simulink model "Parametrica"  (R2020b)
settings: Solver=VariableStepAuto  StartTime=0.0  StopTime=Smi.general.simulation_time  FixedStep=0.001  MaxStep=0.001  RelTol=1e-3  AbsTol=1e-3  EnableMultiTasking=on
undefined symbols (not defined in the file or in its folder): Smi, X, Y, Z
libraries: sm_lib x755, nesl_utility x196, simulink x8, dspsrcs4 x8, cstblocks x8
(part 25 of 26)

== system Parametrica/MOVING CHASSIS/RR SUSPENSION/PUSHROD ==
  Cylindrical Solid : sm_lib/Body Elements/Cylindrical Solid  GraphicAmbientColor=[0.15 0.15 0.15 1.0]  BasedOnType=Density  CenterOfMass=[0 0 0]  CenterOfMassUnits=m  GraphicDiffuseColor=[0.8 0.6 0.0]  CylinderLength=Smi.Car.REAR.RIGHT.Dimension.Pushrod  CylinderLengthUnits=mm  CylinderRadius=Smi.Graphic.radius_links  CylinderRadiusUnits=mm  Density=1000  DensityUnits=kg/m^3  DoExposeReferenceFrame=off  GraphicEmissiveColor=[0.0 0.0 0.0 1.0]  ExportEntireGeometry=off  SerializedFrames=<Frames><Frame><Id>Frame1</Id><Value><Name>F1</Name><Origin><Source>GeometricFeature</Source><FeatureName>top surface</FeatureName></Origin><PrimaryAxis><DefinedDirection>+Z</DefinedDirection><Source>ReferenceFrame</Source><SourceDirection>+Z</SourceDirection><FeatureName></FeatureName></PrimaryAxis><SecondaryAxis><DefinedDirection>+X</DefinedDirection><Source>ReferenceFrame</Source><SourceDirection>+X</SourceDirection><FeatureName></FeatureName></SecondaryAxis></Value></Frame><Frame><Id>Frame2</Id><Value><Name>F2</Name><Origin><Source>GeometricFeature</Source><FeatureName>bottom curve</FeatureName></Origin><PrimaryAxis><DefinedDirection>+Z</DefinedDirection><Source>ReferenceFrame</Source><SourceDirection>+Z</SourceDirection><FeatureName></FeatureName></PrimaryAxis><SecondaryAxis><DefinedDirection>+X</DefinedDirection><Source>ReferenceFrame</Source><SourceDirection>+X</SourceDirection><FeatureName></FeatureName></SecondaryAxis></Value></Frame></Frames>  MarkerShape=Sphere  MarkerSize=10  GraphicType=FromGeometry  InertiaType=CalculateFromGeometry  Mass=1  MassUnits=kg  MomentsOfInertia=[1 1 1]  MomentsOfInertiaUnits=kg*m^2  GraphicOpacity=1.0  ProductsOfInertia=[0 0 0]  ProductsOfInertiaUnits=kg*m^2  GraphicShininess=75  GraphicSpecularColor=[0.5 0.5 0.5 1.0]  GraphicVisPropType=SimpleVisualProperties
  Spherical Solid : sm_lib/Body Elements/Spherical Solid  GraphicAmbientColor=[0.15 0.15 0.15 1.0]  BasedOnType=Density  CenterOfMass=[0 0 0]  CenterOfMassUnits=m  GraphicDiffuseColor=[0.8 0.6 0.0]  Density=0  DensityUnits=kg/m^3  DoExposeReferenceFrame=on  GraphicEmissiveColor=[0.0 0.0 0.0 1.0]  ExportEntireGeometry=off  SerializedExposedGeometries=<ExposedGeometries/>  SerializedFrames=<Frames/>  MarkerShape=Sphere  MarkerSize=10  GraphicType=FromGeometry  InertiaType=CalculateFromGeometry  Mass=1  MassUnits=kg  MomentsOfInertia=[1 1 1]  MomentsOfInertiaUnits=kg*m^2  GraphicOpacity=1.0  ProductsOfInertia=[0 0 0]  ProductsOfInertiaUnits=kg*m^2  GraphicShininess=75  GraphicSpecularColor=[0.5 0.5 0.5 1.0]  SphereRadius=Smi.Graphic.radius_spheres  SphereRadiusUnits=mm  GraphicVisPropType=SimpleVisualProperties
  Spherical Solid1 : sm_lib/Body Elements/Spherical Solid  GraphicAmbientColor=[0.15 0.15 0.15 1.0]  BasedOnType=Density  CenterOfMass=[0 0 0]  CenterOfMassUnits=m  GraphicDiffuseColor=[0.8 0.6 0.0]  Density=0  DensityUnits=kg/m^3  DoExposeReferenceFrame=on  GraphicEmissiveColor=[0.0 0.0 0.0 1.0]  ExportEntireGeometry=off  SerializedExposedGeometries=<ExposedGeometries/>  SerializedFrames=<Frames/>  MarkerShape=Sphere  MarkerSize=10  GraphicType=FromGeometry  InertiaType=CalculateFromGeometry  Mass=1  MassUnits=kg  MomentsOfInertia=[1 1 1]  MomentsOfInertiaUnits=kg*m^2  GraphicOpacity=1.0  ProductsOfInertia=[0 0 0]  ProductsOfInertiaUnits=kg*m^2  GraphicShininess=75  GraphicSpecularColor=[0.5 0.5 0.5 1.0]  SphereRadius=Smi.Graphic.radius_spheres  SphereRadiusUnits=mm  GraphicVisPropType=SimpleVisualProperties
  CRANK : PMIOPort  Side=Left
  UPPER WISHBONE : PMIOPort  Port=2  Side=Right
  connections:
  Cylindrical Solid/RConn1 -- Spherical Solid/RConn1 -- CRANK/RConn1
  Spherical Solid1/RConn1 -- UPPER WISHBONE/RConn1 -- Cylindrical Solid/LConn1

== system Parametrica/MOVING CHASSIS/RR SUSPENSION/STEM ==
  ATTACCO STEM : sm_lib/Body Elements/Extruded Solid  GraphicAmbientColor=[0.15 0.15 0.15 1.0]  BasedOnType=Density  CenterOfMass=[0 0 0]  CenterOfMassUnits=m  GraphicDiffuseColor=[1.0 0.0 0.2]  ExportConvexHullGeometry=off  ExtrusionCrossSection=[0 0; 22 0; 20 22; 2 22]  ExtrusionCrossSectionUnits=mm  Density=1000  DensityUnits=kg/m^3  DoExposeReferenceFrame=off  GraphicEmissiveColor=[0.0 0.0 0.0 1.0]  ExportEntireGeometry=off  ExtrusionLength=5  ExtrusionLengthUnits=mm  ExtrusionType=General  SerializedFrames=<Frames><Frame><Id>Frame1</Id><Value><Name>F1</Name><Origin><Source>GeometricFeature</Source><FeatureName>side surface 1</FeatureName></Origin><PrimaryAxis><DefinedDirection>+Z</DefinedDirection><Source>ReferenceFrame</Source><SourceDirection>+Y</SourceDirection><FeatureName></FeatureName></PrimaryAxis><SecondaryAxis><DefinedDirection>+X</DefinedDirection><Source>ReferenceFrame</Source><SourceDirection>+X</SourceDirection><FeatureName></FeatureName></SecondaryAxis></Value></Frame><Frame><Id>Frame2</Id><Value><Name>F2</Name><Origin><Source>CenterOfMassFrame</Source><FeatureName></FeatureName></Origin><PrimaryAxis><DefinedDirection>+Y</DefinedDirection><Source>ReferenceFrame</Source><SourceDirection>-Y</SourceDirection><FeatureName></FeatureName></PrimaryAxis><SecondaryAxis><DefinedDirection>+X</DefinedDirection><Source>ReferenceFrame</Source><SourceDirection>+X</SourceDirection><FeatureName></FeatureName></SecondaryAxis></Value></Frame></Frames>  MarkerShape=Sphere  MarkerSize=10  GraphicType=FromGeometry  InertiaType=CalculateFromGeometry  Mass=1  MassUnits=kg  MomentsOfInertia=[1 1 1]  MomentsOfInertiaUnits=kg*m^2  PolygonNumSides=3  GraphicOpacity=1.0  PolygonOuterRadius=1  PolygonOuterRadiusUnits=m  ProductsOfInertia=[0 0 0]  ProductsOfInertiaUnits=kg*m^2  GraphicShininess=75  GraphicSpecularColor=[0.5 0.5 0.5 1.0]  GraphicVisPropType=SimpleVisualProperties
  STEM : sm_lib/Body Elements/Revolved Solid  GraphicAmbientColor=[0.15 0.15 0.15 1.0]  BasedOnType=Density  CenterOfMass=[0 0 0]  CenterOfMassUnits=m  GraphicDiffuseColor=[1.0 0.0 0.2]  ExportConvexHullGeometry=off  Density=1000  DensityUnits=kg/m^3  DoExposeReferenceFrame=on  GraphicEmissiveColor=[0.0 0.0 0.0 1.0]  ExportEntireGeometry=off  SerializedFrames=<Frames><Frame><Id>Frame1</Id><Value><Name>F1</Name><Origin><Source>GeometricFeature</Source><FeatureName>side surface 5</FeatureName></Origin><PrimaryAxis><DefinedDirection>+Z</DefinedDirection><Source>ReferenceFrame</Source><SourceDirection>+Z</SourceDirection><FeatureName></FeatureName></PrimaryAxis><SecondaryAxis><DefinedDirection>+X</DefinedDirection><Source>ReferenceFrame</Source><SourceDirection>+X</SourceDirection><FeatureName></FeatureName></SecondaryAxis></Value></Frame></Frames>  MarkerShape=Sphere  MarkerSize=10  GraphicType=FromGeometry  InertiaType=CalculateFromGeometry  Mass=1  MassUnits=kg  MomentsOfInertia=[1 1 1]  MomentsOfInertiaUnits=kg*m^2  GraphicOpacity=1.0  ProductsOfInertia=[0 0 0]  ProductsOfInertiaUnits=kg*m^2  RevolutionCrossSection=[0 0 ; 3 0 ; 3 50 ; 21 50 ; 21 52 ; 0 52]  RevolutionCrossSectionUnits=mm  RevolutionAngle=180  RevolutionAngleUnits=deg  RevolutionExtent=Full  GraphicShininess=75  GraphicSpecularColor=[0.5 0.5 0.5 1.0]  GraphicVisPropType=SimpleVisualProperties
  CRANK : PMIOPort  Side=Left
  AMMO : PMIOPort  Port=2  Side=Right
  connections:
  ATTACCO STEM/LConn1 -- STEM/LConn1
  ATTACCO STEM/RConn1 -- CRANK/RConn1
  STEM/RConn1 -- AMMO/RConn1

== system Parametrica/MOVING CHASSIS/RR SUSPENSION/TIE ROD ==
  Cylindrical Solid : sm_lib/Body Elements/Cylindrical Solid  GraphicAmbientColor=[0.15 0.15 0.15 1.0]  BasedOnType=Density  CenterOfMass=[0 0 0]  CenterOfMassUnits=m  GraphicDiffuseColor=[1.0 0.6 0.4]  CylinderLength=Smi.Car.REAR.RIGHT.Dimension.Tie_rod  CylinderLengthUnits=mm  CylinderRadius=Smi.Graphic.radius_links  CylinderRadiusUnits=mm  Density=1000  DensityUnits=kg/m^3  DoExposeReferenceFrame=off  GraphicEmissiveColor=[0.0 0.0 0.0 1.0]  ExportEntireGeometry=off  SerializedFrames=<Frames><Frame><Id>Frame1</Id><Value><Name>F1</Name><Origin><Source>GeometricFeature</Source><FeatureName>top surface</FeatureName></Origin><PrimaryAxis><DefinedDirection>+Z</DefinedDirection><Source>ReferenceFrame</Source><SourceDirection>+Z</SourceDirection><FeatureName></FeatureName></PrimaryAxis><SecondaryAxis><DefinedDirection>+X</DefinedDirection><Source>ReferenceFrame</Source><SourceDirection>+X</SourceDirection><FeatureName></FeatureName></SecondaryAxis></Value></Frame><Frame><Id>Frame2</Id><Value><Name>F2</Name><Origin><Source>GeometricFeature</Source><FeatureName>bottom curve</FeatureName></Origin><PrimaryAxis><DefinedDirection>+Z</DefinedDirection><Source>ReferenceFrame</Source><SourceDirection>+Z</SourceDirection><FeatureName></FeatureName></PrimaryAxis><SecondaryAxis><DefinedDirection>+X</DefinedDirection><Source>ReferenceFrame</Source><SourceDirection>+X</SourceDirection><FeatureName></FeatureName></SecondaryAxis></Value></Frame></Frames>  MarkerShape=Sphere  MarkerSize=10  GraphicType=FromGeometry  InertiaType=CalculateFromGeometry  Mass=1  MassUnits=kg  MomentsOfInertia=[1 1 1]  MomentsOfInertiaUnits=kg*m^2  GraphicOpacity=1.0  ProductsOfInertia=[0 0 0]  ProductsOfInertiaUnits=kg*m^2  GraphicShininess=75  GraphicSpecularColor=[0.5 0.5 0.5 1.0]  GraphicVisPropType=SimpleVisualProperties
  Spherical Solid : sm_lib/Body Elements/Spherical Solid  GraphicAmbientColor=[0.15 0.15 0.15 1.0]  BasedOnType=Density  CenterOfMass=[0 0 0]  CenterOfMassUnits=m  GraphicDiffuseColor=[1.0 0.6 0.4]  Density=0  DensityUnits=kg/m^3  DoExposeReferenceFrame=on  GraphicEmissiveColor=[0.0 0.0 0.0 1.0]  ExportEntireGeometry=off  SerializedExposedGeometries=<ExposedGeometries/>  SerializedFrames=<Frames/>  MarkerShape=Sphere  MarkerSize=10  GraphicType=FromGeometry  InertiaType=CalculateFromGeometry  Mass=1  MassUnits=kg  MomentsOfInertia=[1 1 1]  MomentsOfInertiaUnits=kg*m^2  GraphicOpacity=1.0  ProductsOfInertia=[0 0 0]  ProductsOfInertiaUnits=kg*m^2  GraphicShininess=75  GraphicSpecularColor=[0.5 0.5 0.5 1.0]  SphereRadius=Smi.Graphic.radius_spheres  SphereRadiusUnits=mm  GraphicVisPropType=SimpleVisualProperties
  Spherical Solid1 : sm_lib/Body Elements/Spherical Solid  GraphicAmbientColor=[0.15 0.15 0.15 1.0]  BasedOnType=Density  CenterOfMass=[0 0 0]  CenterOfMassUnits=m  GraphicDiffuseColor=[1.0 0.6 0.4]  Density=0  DensityUnits=kg/m^3  DoExposeReferenceFrame=on  GraphicEmissiveColor=[0.0 0.0 0.0 1.0]  ExportEntireGeometry=off  SerializedExposedGeometries=<ExposedGeometries/>  SerializedFrames=<Frames/>  MarkerShape=Sphere  MarkerSize=10  GraphicType=FromGeometry  InertiaType=CalculateFromGeometry  Mass=1  MassUnits=kg  MomentsOfInertia=[1 1 1]  MomentsOfInertiaUnits=kg*m^2  GraphicOpacity=1.0  ProductsOfInertia=[0 0 0]  ProductsOfInertiaUnits=kg*m^2  GraphicShininess=75  GraphicSpecularColor=[0.5 0.5 0.5 1.0]  SphereRadius=Smi.Graphic.radius_spheres  SphereRadiusUnits=mm  GraphicVisPropType=SimpleVisualProperties
  TIE HUB : PMIOPort  Side=Left
  TIE RACK : PMIOPort  Port=2  Side=Right
  connections:
  Cylindrical Solid/RConn1 -- Spherical Solid/RConn1 -- TIE RACK/RConn1
  Spherical Solid1/RConn1 -- TIE HUB/RConn1 -- Cylindrical Solid/LConn1

== system Parametrica/MOVING CHASSIS/RR SUSPENSION/UPPER WISHBONE ==
  A : sm_lib/Body Elements/Spherical Solid  GraphicAmbientColor=[0.15 0.15 0.15 1.0]  BasedOnType=Density  CenterOfMass=[0 0 0]  CenterOfMassUnits=m  GraphicDiffuseColor=[1.0 0.6 0.2]  Density=0  DensityUnits=kg/m^3  DoExposeReferenceFrame=on  GraphicEmissiveColor=[0.0 0.0 0.0 1.0]  ExportEntireGeometry=off  SerializedExposedGeometries=<ExposedGeometries/>  SerializedFrames=<Frames/>  MarkerShape=Sphere  MarkerSize=10  GraphicType=FromGeometry  InertiaType=CalculateFromGeometry  Mass=1  MassUnits=kg  MomentsOfInertia=[1 1 1]  MomentsOfInertiaUnits=kg*m^2  GraphicOpacity=1.0  ProductsOfInertia=[0 0 0]  ProductsOfInertiaUnits=kg*m^2  GraphicShininess=75  GraphicSpecularColor=[0.5 0.5 0.5 1.0]  SphereRadius=Smi.Graphic.radius_spheres  SphereRadiusUnits=mm  GraphicVisPropType=SimpleVisualProperties
  A-B : sm_lib/Frames and Transforms/Rigid Transform  TranslationMethod=None  TranslationStandardOffset=0  TranslationLengthUnit=mm  TranslationStandardAxis=+Z  TranslationCartesianOffset=Smi.Car.FRONT.LEFT.A  TranslationROffset=0  TranslationROffsetUnits=m  TranslationZOffset=0  TranslationZOffsetUnits=m  TranslationThetaOffset=0  TranslationThetaOffsetUnits=deg  RotationMethod=StandardAxis  RotationAngleUnits=rad  RotationStandardAxis=+Z  RotationAngle=-Smi.Car.REAR.RIGHT.Dimension.plane_UW.wish_angle  RotationArbitraryAxis=[0 0 1]  FollAlignAxisA=+X  BaseAlignAxisA=+Y  FollAlignAxisB=+Y  BaseAlignAxisB=+Z  RotationSequenceAxes=FollowerAxes  RotationSequence=XYZ  RotationSequenceAngles=0  RotationSequenceAnglesUnits=rad  RotationMatrix=[1 0 0; 0 1 0; 0 0 1]
      settings: SourceProductName=Multibody
  A-PS : sm_lib/Frames and Transforms/Rigid Transform  TranslationMethod=Cartesian  TranslationStandardOffset=0  TranslationLengthUnit=mm  TranslationStandardAxis=+Z  TranslationCartesianOffset=Smi.Car.REAR.RIGHT.Dimension.plane_UW.PS_t_coord-Smi.Car.REAR.RIGHT.Dimension.plane_UW.A_t_coord  TranslationROffset=0  TranslationROffsetUnits=m  TranslationZOffset=0  TranslationZOffsetUnits=m  TranslationThetaOffset=0  TranslationThetaOffsetUnits=deg  RotationMethod=None  RotationAngleUnits=deg  RotationStandardAxis=+Z  RotationAngle=0.0  RotationArbitraryAxis=[0 0 1]  FollAlignAxisA=+X  BaseAlignAxisA=+Y  FollAlignAxisB=+Y  BaseAlignAxisB=+Z  RotationSequenceAxes=FollowerAxes  RotationSequence=XYZ  RotationSequenceAngles=0  RotationSequenceAnglesUnits=rad  RotationMatrix=[1 0 0; 0 1 0; 0 0 1]
      settings: SourceProductName=Multibody
  B : sm_lib/Body Elements/Spherical Solid  GraphicAmbientColor=[0.15 0.15 0.15 1.0]  BasedOnType=Density  CenterOfMass=[0 0 0]  CenterOfMassUnits=m  GraphicDiffuseColor=[1.0 0.6 0.2]  Density=0  DensityUnits=kg/m^3  DoExposeReferenceFrame=on  GraphicEmissiveColor=[0.0 0.0 0.0 1.0]  ExportEntireGeometry=off  SerializedExposedGeometries=<ExposedGeometries/>  SerializedFrames=<Frames/>  MarkerShape=Sphere  MarkerSize=10  GraphicType=FromGeometry  InertiaType=CalculateFromGeometry  Mass=1  MassUnits=kg  MomentsOfInertia=[1 1 1]  MomentsOfInertiaUnits=kg*m^2  GraphicOpacity=1.0  ProductsOfInertia=[0 0 0]  ProductsOfInertiaUnits=kg*m^2  GraphicShininess=75  GraphicSpecularColor=[0.5 0.5 0.5 1.0]  SphereRadius=Smi.Graphic.radius_spheres  SphereRadiusUnits=mm  GraphicVisPropType=SimpleVisualProperties
  INNER CYL : sm_lib/Body Elements/Cylindrical Solid  GraphicAmbientColor=[0.15 0.15 0.15 1.0]  BasedOnType=Density  CenterOfMass=[0 0 0]  CenterOfMassUnits=m  GraphicDiffuseColor=[1.0 0.6 0.2]  CylinderLength=Smi.Car.REAR.RIGHT.Dimension.inner_cyl_UW  CylinderLengthUnits=mm  CylinderRadius=Smi.Graphic.radius_links  CylinderRadiusUnits=mm  Density=1000  DensityUnits=kg/m^3  DoExposeReferenceFrame=off  GraphicEmissiveColor=[0.0 0.0 0.0 1.0]  ExportEntireGeometry=off  SerializedFrames=<Frames><Frame><Id>Frame3</Id><Value><Name>F1</Name><Origin><Source>GeometricFeature</Source><FeatureName>top curve</FeatureName></Origin><PrimaryAxis><DefinedDirection>+Z</DefinedDirection><Source>ReferenceFrame</Source><SourceDirection>+Y</SourceDirection><FeatureName></FeatureName></PrimaryAxis><SecondaryAxis><DefinedDirection>+X</DefinedDirection><Source>ReferenceFrame</Source><SourceDirection>+X</SourceDirection><FeatureName></FeatureName></SecondaryAxis></Value></Frame><Frame><Id>Frame4</Id><Value><Name>F4</Name><Origin><Source>GeometricFeature</Source><FeatureName>bottom surface</FeatureName></Origin><PrimaryAxis><DefinedDirection>+Z</DefinedDirection><Source>ReferenceFrame</Source><SourceDirection>+X</SourceDirection><FeatureName></FeatureName></PrimaryAxis><SecondaryAxis><DefinedDirection>+X</DefinedDirection><Source>ReferenceFrame</Source><SourceDirection>+Y</SourceDirection><FeatureName></FeatureName></SecondaryAxis></Value></Frame></Frames>  MarkerShape=Sphere  MarkerSize=10  GraphicType=FromGeometry  InertiaType=CalculateFromGeometry  Mass=1  MassUnits=kg  MomentsOfInertia=[1 1 1]  MomentsOfInertiaUnits=kg*m^2  GraphicOpacity=1.0  ProductsOfInertia=[0 0 0]  ProductsOfInertiaUnits=kg*m^2  GraphicShininess=75  GraphicSpecularColor=[0.5 0.5 0.5 1.0]  GraphicVisPropType=SimpleVisualProperties
  OUTER CYL : sm_lib/Body Elements/Cylindrical Solid  GraphicAmbientColor=[0.15 0.15 0.15 1.0]  BasedOnType=Density  CenterOfMass=[0 0 0]  CenterOfMassUnits=m  GraphicDiffuseColor=[1.0 0.6 0.2]  CylinderLength=Smi.Car.REAR.RIGHT.Dimension.outer_cyl_UW  CylinderLengthUnits=mm  CylinderRadius=Smi.Graphic.radius_links  CylinderRadiusUnits=mm  Density=1000  DensityUnits=kg/m^3  DoExposeReferenceFrame=off  GraphicEmissiveColor=[0.0 0.0 0.0 1.0]  ExportEntireGeometry=off  SerializedFrames=<Frames><Frame><Id>Frame1</Id><Value><Name>F1</Name><Origin><Source>GeometricFeature</Source><FeatureName>top surface</FeatureName></Origin><PrimaryAxis><DefinedDirection>+Y</DefinedDirection><Source>ReferenceFrame</Source><SourceDirection>+Z</SourceDirection><FeatureName></FeatureName></PrimaryAxis><SecondaryAxis><DefinedDirection>+X</DefinedDirection><Source>ReferenceFrame</Source><SourceDirection>+X</SourceDirection><FeatureName></FeatureName></SecondaryAxis></Value></Frame><Frame><Id>Frame2</Id><Value><Name>F2</Name><Origin><Source>GeometricFeature</Source><FeatureName>bottom surface</FeatureName></Origin><PrimaryAxis><DefinedDirection>+Y</DefinedDirection><Source>ReferenceFrame</Source><SourceDirection>+Z</SourceDirection><FeatureName></FeatureName></PrimaryAxis><SecondaryAxis><DefinedDirection>+X</DefinedDirection><Source>ReferenceFrame</Source><SourceDirection>+X</SourceDirection><FeatureName></FeatureName></SecondaryAxis></Value></Frame></Frames>  MarkerShape=Sphere  MarkerSize=10  GraphicType=FromGeometry  InertiaType=CalculateFromGeometry  Mass=1  MassUnits=kg  MomentsOfInertia=[1 1 1]  MomentsOfInertiaUnits=kg*m^2  GraphicOpacity=1.0  ProductsOfInertia=[0 0 0]  ProductsOfInertiaUnits=kg*m^2  GraphicShininess=75  GraphicSpecularColor=[0.5 0.5 0.5 1.0]  GraphicVisPropType=SimpleVisualProperties
  UBJ : sm_lib/Body Elements/Spherical Solid  GraphicAmbientColor=[0.15 0.15 0.15 1.0]  BasedOnType=Density  CenterOfMass=[0 0 0]  CenterOfMassUnits=m  GraphicDiffuseColor=[1.0 0.6 0.2]  Density=1000  DensityUnits=kg/m^3  DoExposeReferenceFrame=on  GraphicEmissiveColor=[0.0 0.0 0.0 1.0]  ExportEntireGeometry=off  SerializedExposedGeometries=<ExposedGeometries/>  SerializedFrames=<Frames/>  MarkerShape=Sphere  MarkerSize=10  GraphicType=FromGeometry  InertiaType=CalculateFromGeometry  Mass=1  MassUnits=kg  MomentsOfInertia=[1 1 1]  MomentsOfInertiaUnits=kg*m^2  GraphicOpacity=1.0  ProductsOfInertia=[0 0 0]  ProductsOfInertiaUnits=kg*m^2  GraphicShininess=75  GraphicSpecularColor=[0.5 0.5 0.5 1.0]  SphereRadius=Smi.Graphic.radius_spheres  SphereRadiusUnits=mm  GraphicVisPropType=SimpleVisualProperties
  A UCS : PMIOPort  Side=Left
  B UCS : PMIOPort  Port=2  Side=Left
  PUSHROD UCS : PMIOPort  Port=3  Side=Right
  UBJ UCS : PMIOPort  Port=4  Side=Right
  connections:
  A UCS/RConn1 -- OUTER CYL/RConn1 -- A-PS/LConn1 -- A/RConn1
  UBJ UCS/RConn1 -- UBJ/RConn1 -- OUTER CYL/LConn1 -- A-B/LConn1
  B UCS/RConn1 -- B/RConn1 -- INNER CYL/LConn1
  A-B/RConn1 -- INNER CYL/RConn1
  A-PS/RConn1 -- PUSHROD UCS/RConn1

== system Parametrica/MOVING CHASSIS/RR SUSPENSION/WHEEL ==
  Revolved Solid : sm_lib/Body Elements/Revolved Solid  Commented=on  GraphicAmbientColor=[0.15 0.15 0.15 1.0]  BasedOnType=Density  CenterOfMass=[0 0 0]  CenterOfMassUnits=m  GraphicDiffuseColor=[0.8 1.0 0.8]  ExportConvexHullGeometry=off  Density=1000  DensityUnits=kg/m^3  DoExposeReferenceFrame=off  GraphicEmissiveColor=[0.0 0.0 0.0 1.0]  ExportEntireGeometry=off  SerializedFrames=<Frames><Frame><Id>Frame1</Id><Value><Name>F1</Name><Origin><Source>ReferenceFrame</Source><FeatureName></FeatureName></Origin><PrimaryAxis><DefinedDirection>+Z</DefinedDirection><Source>ReferenceFrame</Source><SourceDirection>+Y</SourceDirection><FeatureName></FeatureName></PrimaryAxis><SecondaryAxis><DefinedDirection>+X</DefinedDirection><Source>ReferenceFrame</Source><SourceDirection>-X</SourceDirection><FeatureName></FeatureName></SecondaryAxis></Value></Frame></Frames>  MarkerShape=Sphere  MarkerSize=10  GraphicType=FromGeometry  InertiaType=CalculateFromGeometry  Mass=1  MassUnits=kg  MomentsOfInertia=[1 1 1]  MomentsOfInertiaUnits=kg*m^2  GraphicOpacity=0.5  ProductsOfInertia=[0 0 0]  ProductsOfInertiaUnits=kg*m^2  RevolutionCrossSection=Smi.Car.FRONT.LEFT.Dimension.tyre_profile  RevolutionCrossSectionUnits=mm  RevolutionAngle=180  RevolutionAngleUnits=deg  RevolutionExtent=Full  GraphicShininess=75  GraphicSpecularColor=[0.5 0.5 0.5 1.0]  GraphicVisPropType=SimpleVisualProperties
  Rigid Transform : sm_lib/Frames and Transforms/Rigid Transform  TranslationMethod=StandardAxis  TranslationStandardOffset=Smi.Car.REAR.RIGHT.TYRE_DIAMETER/2+3  TranslationLengthUnit=mm  TranslationStandardAxis=-Z  TranslationCartesianOffset=[0 0 0]  TranslationROffset=0  TranslationROffsetUnits=m  TranslationZOffset=0  TranslationZOffsetUnits=m  TranslationThetaOffset=0  TranslationThetaOffsetUnits=deg  RotationMethod=None  RotationAngleUnits=deg  RotationStandardAxis=+Z  RotationAngle=0.0  RotationArbitraryAxis=[0 0 1]  FollAlignAxisA=+X  BaseAlignAxisA=+Y  FollAlignAxisB=+Y  BaseAlignAxisB=+Z  RotationSequenceAxes=FollowerAxes  RotationSequence=XYX  RotationSequenceAngles=[0 0 0]  RotationSequenceAnglesUnits=deg  RotationMatrix=[1 0 0; 0 1 0; 0 0 1]
  Spherical Solid : sm_lib/Body Elements/Spherical Solid  Commented=on  GraphicAmbientColor=[0.15 0.15 0.15 1.0]  BasedOnType=Density  CenterOfMass=[0 0 0]  CenterOfMassUnits=m  GraphicDiffuseColor=[1.0 0.0 0.2]  Density=0  DensityUnits=kg/m^3  DoExposeReferenceFrame=on  GraphicEmissiveColor=[0.0 0.0 0.0 1.0]  ExportEntireGeometry=on  SerializedExposedGeometries=<ExposedGeometries><ExposedGeometry><RawGeometryId>entire</RawGeometryId><ExposedGeometryId>G</ExposedGeometryId></ExposedGeometry></ExposedGeometries>  SerializedFrames=<Frames/>  MarkerShape=Sphere  MarkerSize=10  GraphicType=FromGeometry  InertiaType=CalculateFromGeometry  Mass=1  MassUnits=kg  MomentsOfInertia=[1 1 1]  MomentsOfInertiaUnits=kg*m^2  GraphicOpacity=0  ProductsOfInertia=[0 0 0]  ProductsOfInertiaUnits=kg*m^2  GraphicShininess=75  GraphicSpecularColor=[0.5 0.5 0.5 1.0]  SphereRadius=Smi.Car.FRONT.LEFT.TYRE_DIAMETER/2  SphereRadiusUnits=mm  GraphicVisPropType=SimpleVisualProperties
  TIRE : sm_lib/Body Elements/File Solid  ExtGeomFileName=Parameters\tire.stp  UnitType=FromFile  ExtGeomFileUnits=m  StepReaderType=HEX  ExportConvexHullGeometry=on  InertiaType=PointMass  Mass=1  MassUnits=kg  CenterOfMass=[0 0 0]  CenterOfMassUnits=m  MomentsOfInertia=[1 1 1]  MomentsOfInertiaUnits=kg*m^2  ProductsOfInertia=[0 0 0]  ProductsOfInertiaUnits=kg*m^2  BasedOnType=DensityFromFile  Density=1000  DensityUnits=kg/m^3  DoExposeReferenceFrame=off  SerializedFrames=<Frames><Frame><Id>Frame1</Id><Value><Name>F1</Name><Origin><Source>ReferenceFrame</Source><FeatureName></FeatureName></Origin><PrimaryAxis><DefinedDirection>+Z</DefinedDirection><Source>ReferenceFrame</Source><SourceDirection>+Z</SourceDirection><FeatureName></FeatureName></PrimaryAxis><SecondaryAxis><DefinedDirection>+X</DefinedDirection><Source>ReferenceFrame</Source><SourceDirection>+Y</SourceDirection><FeatureName></FeatureName></SecondaryAxis></Value></Frame></Frames>  GraphicType=FromGeometry  MarkerShape=Sphere  MarkerSize=10  GraphicVisPropType=SimpleVisualProperties  GraphicDiffuseColor=[0.5 0.5 0.5]  GraphicSpecularColor=[0.5 0.5 0.5 1.0]  GraphicAmbientColor=[0.15 0.15 0.15 1.0]  GraphicEmissiveColor=[0.0 0.0 0.0 1.0]  GraphicShininess=75  GraphicOpacity=1.0
  WC : PMIOPort  Side=Left
  Contact Sphere : PMIOPort  Port=2  Side=Right
  CP REAL : PMIOPort  Port=3  Side=Right
  connections:
  Spherical Solid/RConn1 -- Rigid Transform/LConn1 -- TIRE/LConn1 -- WC/RConn1
  CP REAL/RConn1 -- Rigid Transform/RConn1
  Contact Sphere/RConn1 -- TIRE/RConn1

== system Parametrica/MOVING CHASSIS/RR SUSPENSION/Wheel Angle Sensing ==
  Gain : Gain  Gain=-1
  PS-Simulink Converter : nesl_utility/PS-Simulink Converter  PhysicalDomain=network_engine_domain  SubClassName=ps_output  LeftPortType=input  RightPortType=output  PseudoPeriodic=off  Frequencies=[]  Unit=deg  AffineConversion=off
  PS-Simulink Converter1 : nesl_utility/PS-Simulink Converter  PhysicalDomain=network_engine_domain  SubClassName=ps_output  LeftPortType=input  RightPortType=output  PseudoPeriodic=off  Frequencies=[]  Unit=inherit  AffineConversion=off
  PS-Simulink Converter2 : nesl_utility/PS-Simulink Converter  PhysicalDomain=network_engine_domain  SubClassName=ps_output  LeftPortType=input  RightPortType=output  PseudoPeriodic=off  Frequencies=[]  Unit=deg  AffineConversion=off
  PS-Simulink Converter3 : nesl_utility/PS-Simulink Converter  PhysicalDomain=network_engine_domain  SubClassName=ps_output  LeftPortType=input  RightPortType=output  PseudoPeriodic=off  Frequencies=[]  Unit=inherit  AffineConversion=off
  Product : Product
  Product1 : Product
  Scope : Scope
  Scope1 : Scope
  Selector : Selector  InputPortWidth=3  IndexOptions=Index vector (dialog)  Indices=[1]  OutputSizes=1
  Selector1 : Selector  InputPortWidth=3  IndexOptions=Index vector (dialog)  Indices=[3]  OutputSizes=1
  To Workspace : ToWorkspace  VariableName=RR_camber  SaveFormat=Timeseries  SampleTime=-1
  To Workspace1 : ToWorkspace  VariableName=RR_toe  SaveFormat=Timeseries  SampleTime=-1
  Transform Sensor : sm_lib/Frames and Transforms/Transform Sensor  MeasurementFrame=Base  SenseAngle=on  SenseAxis=on  SenseAngle1=off  SenseAngle2=off  SenseAngle3=off  SenseQ=off  SenseR=off  SenseOmegaX=off  SenseOmegaY=off  SenseOmegaZ=off  SenseOmega1=off  SenseOmega2=off  SenseOmega3=off  SenseQDot=off  SenseRDot=off  SenseAlphaX=off  SenseAlphaY=off  SenseAlphaZ=off  SenseAlpha1=off  SenseAlpha2=off  SenseAlpha3=off  SenseQDDot=off  SenseRDDot=off  SenseX=off  SenseY=off  SenseZ=off  SenseRad=off  SenseAzim=off  SenseDist=off  SenseInc=off  SenseXDot=off  SenseYDot=off  SenseZDot=off  SenseRadDot=off  SenseAzimDot=off  SenseDistDot=off  SenseIncDot=off  SenseXDDot=off  SenseYDDot=off  SenseZDDot=off  SenseRadDDot=off  SenseAzimDDot=off  SenseDistDDot=off  SenseIncDDot=off
  Transform Sensor1 : sm_lib/Frames and Transforms/Transform Sensor  MeasurementFrame=Base  SenseAngle=on  SenseAxis=on  SenseAngle1=off  SenseAngle2=off  SenseAngle3=off  SenseQ=off  SenseR=off  SenseOmegaX=off  SenseOmegaY=off  SenseOmegaZ=off  SenseOmega1=off  SenseOmega2=off  SenseOmega3=off  SenseQDot=off  SenseRDot=off  SenseAlphaX=off  SenseAlphaY=off  SenseAlphaZ=off  SenseAlpha1=off  SenseAlpha2=off  SenseAlpha3=off  SenseQDDot=off  SenseRDDot=off  SenseX=off  SenseY=off  SenseZ=off  SenseRad=off  SenseAzim=off  SenseDist=off  SenseInc=off  SenseXDot=off  SenseYDot=off  SenseZDot=off  SenseRadDot=off  SenseAzimDot=off  SenseDistDot=off  SenseIncDot=off  SenseXDDot=off  SenseYDDot=off  SenseZDDot=off  SenseRadDDot=off  SenseAzimDDot=off  SenseDistDDot=off  SenseIncDDot=off
  WHEEL : PMIOPort  Side=Left
  WORLD : PMIOPort  Port=2  Side=Right
  wires:
  Product/1 -> To Workspace/1, Scope/1
  PS-Simulink Converter/1 -> Product/1
  Selector1/1 -> Product1/2
  PS-Simulink Converter2/1 -> Gain/1
  Selector/1 -> Product/2
  Product1/1 -> To Workspace1/1, Scope1/1
  PS-Simulink Converter1/1 -> Selector/1
  PS-Simulink Converter3/1 -> Selector1/1
  Gain/1 -> Product1/1
  connections:
  PS-Simulink Converter2/LConn1 -- Transform Sensor1/RConn2
  PS-Simulink Converter/LConn1 -- Transform Sensor/RConn2
  Transform Sensor/RConn1 -- Transform Sensor1/RConn1 -- WORLD/RConn1
  Transform Sensor1/LConn1 -- Transform Sensor/LConn1 -- WHEEL/RConn1
  PS-Simulink Converter3/LConn1 -- Transform Sensor1/RConn3
  PS-Simulink Converter1/LConn1 -- Transform Sensor/RConn3

== system Parametrica/FIXED CHASSIS/ACTUATOR FL/ACTUATOR IN//OUT/Random sine waves ==
  Clock : Clock
  Constant : Constant  Value=Smi.general.random_harshness
  Constant1 : Constant  Value=-100
  Divide : Product  Inputs=*/
  First Order Hold : FirstOrderHold  InitialOutput=-100  ErrorTolerance=30  AllowContinuousInput=on
  Gain : Gain  Gain=100
  Random Source : dspsrcs4/Random Source  SrcType=Uniform  NormMethod=Ziggurat  CltLength=12  MinVal=-Smi.general.random_amplitude*0.5  MaxVal=Smi.general.random_amplitude*0.5  MeanVal=0  VarVal=1  RepMode=Not repeatable  rawSeed=1  IsInherit=off  SampMode=Discrete  SampTime=0.05  SampFrame=1  DataType=Double  OutComplex=Real  OutputFrames=off
  Rate Transition : RateTransition  OutPortSampleTime=0
  Sum : Sum  Inputs=|+-
  Switch : Switch  Criteria=u2 ~= 0
  Varying Lowpass Filter : cstblocks/Linear Parameter Varying/Varying Lowpass Filter  N=5
  f : Outport
  wires:
  Constant/1 -> Varying Lowpass Filter/2
  Random Source/1 -> Rate Transition/1
  Divide/1 -> Gain/1
  Gain/1 -> Sum/2
  Varying Lowpass Filter/1 -> First Order Hold/1
  First Order Hold/1 -> Sum/1
  Clock/1 -> Divide/2, Switch/2, Divide/1
  Sum/1 -> Switch/1
  Constant1/1 -> Switch/3
  Switch/1 -> f/1
  Rate Transition/1 -> Varying Lowpass Filter/1

== system Parametrica/FIXED CHASSIS/ACTUATOR FR/ACTUATOR IN//OUT/Random sine waves ==
  Clock : Clock
  Constant : Constant  Value=Smi.general.random_harshness
  Constant1 : Constant  Value=-100
  Divide : Product  Inputs=*/
  First Order Hold : FirstOrderHold  InitialOutput=-100  ErrorTolerance=30  AllowContinuousInput=on
  Gain : Gain  Gain=100
  Random Source : dspsrcs4/Random Source  SrcType=Uniform  NormMethod=Ziggurat  CltLength=12  MinVal=-Smi.general.random_amplitude*0.5  MaxVal=Smi.general.random_amplitude*0.5  MeanVal=0  VarVal=1  RepMode=Specify seed  rawSeed=1  IsInherit=off  SampMode=Discrete  SampTime=0.05  SampFrame=1  DataType=Double  OutComplex=Real  OutputFrames=off
  Rate Transition : RateTransition  OutPortSampleTime=0
  Sum : Sum  Inputs=|+-
  Switch : Switch  Criteria=u2 ~= 0
  Varying Lowpass Filter : cstblocks/Linear Parameter Varying/Varying Lowpass Filter  N=5
  f : Outport
  wires:
  Constant/1 -> Varying Lowpass Filter/2
  Random Source/1 -> Rate Transition/1
  Divide/1 -> Gain/1
  Gain/1 -> Sum/2
  Varying Lowpass Filter/1 -> First Order Hold/1
  First Order Hold/1 -> Sum/1
  Clock/1 -> Divide/2, Switch/2, Divide/1
  Sum/1 -> Switch/1
  Constant1/1 -> Switch/3
  Switch/1 -> f/1
  Rate Transition/1 -> Varying Lowpass Filter/1

== system Parametrica/FIXED CHASSIS/ACTUATOR RL/ACTUATOR IN//OUT/Random sine waves ==
  Clock : Clock
  Constant : Constant  Value=Smi.general.random_harshness
  Constant1 : Constant  Value=-100
  Divide : Product  Inputs=*/
  First Order Hold : FirstOrderHold  InitialOutput=-100  ErrorTolerance=30  AllowContinuousInput=on
  Gain : Gain  Gain=100
  Random Source : dspsrcs4/Random Source  SrcType=Uniform  NormMethod=Ziggurat  CltLength=12  MinVal=-Smi.general.random_amplitude*0.5  MaxVal=Smi.general.random_amplitude*0.5  MeanVal=0  VarVal=1  RepMode=Specify seed  rawSeed=1  IsInherit=off  SampMode=Discrete  SampTime=0.05  SampFrame=1  DataType=Double  OutComplex=Real  OutputFrames=off
  Rate Transition : RateTransition  OutPortSampleTime=0
  Sum : Sum  Inputs=|+-
  Switch : Switch  Criteria=u2 ~= 0
  Varying Lowpass Filter : cstblocks/Linear Parameter Varying/Varying Lowpass Filter  N=5
  f : Outport
  wires:
  Constant/1 -> Varying Lowpass Filter/2
  Random Source/1 -> Rate Transition/1
  Divide/1 -> Gain/1
  Gain/1 -> Sum/2
  Varying Lowpass Filter/1 -> First Order Hold/1
  First Order Hold/1 -> Sum/1
  Clock/1 -> Divide/2, Switch/2, Divide/1
  Sum/1 -> Switch/1
  Constant1/1 -> Switch/3
  Switch/1 -> f/1
  Rate Transition/1 -> Varying Lowpass Filter/1

== system Parametrica/FIXED CHASSIS/ACTUATOR RR/ACTUATOR IN//OUT/Random sine waves ==
  Clock : Clock
  Constant : Constant  Value=Smi.general.random_harshness
  Constant1 : Constant  Value=-100
  Divide : Product  Inputs=*/
  First Order Hold : FirstOrderHold  InitialOutput=-100  ErrorTolerance=30  AllowContinuousInput=on
  Gain : Gain  Gain=100
  Random Source : dspsrcs4/Random Source  SrcType=Uniform  NormMethod=Ziggurat  CltLength=12  MinVal=-Smi.general.random_amplitude*0.5  MaxVal=Smi.general.random_amplitude*0.5  MeanVal=0  VarVal=1  RepMode=Specify seed  rawSeed=1  IsInherit=off  SampMode=Discrete  SampTime=0.05  SampFrame=1  DataType=Double  OutComplex=Real  OutputFrames=off
  Rate Transition : RateTransition  OutPortSampleTime=0
  Sum : Sum  Inputs=|+-
  Switch : Switch  Criteria=u2 ~= 0
  Varying Lowpass Filter : cstblocks/Linear Parameter Varying/Varying Lowpass Filter  N=5
  f : Outport
  wires:
  Constant/1 -> Varying Lowpass Filter/2
  Random Source/1 -> Rate Transition/1
  Divide/1 -> Gain/1
  Gain/1 -> Sum/2
  Varying Lowpass Filter/1 -> First Order Hold/1
  First Order Hold/1 -> Sum/1
  Clock/1 -> Divide/2, Switch/2, Divide/1
  Sum/1 -> Switch/1
  Constant1/1 -> Switch/3
  Switch/1 -> f/1
  Rate Transition/1 -> Varying Lowpass Filter/1

== system Parametrica/FIXED CHASSIS/BODY/FL HARDPOINTS/A forces sensing ==
  F : Inport
  Demux : Demux  Outputs=3
  To Workspace : ToWorkspace  VariableName=FL_A_Fx  SaveFormat=Timeseries  SampleTime=-1
  To Workspace1 : ToWorkspace  VariableName=FL_A_Fy  SaveFormat=Timeseries  SampleTime=-1
  To Workspace2 : ToWorkspace  VariableName=FL_A_Fz  SaveFormat=Timeseries  SampleTime=-1
  wires:
  Demux/1 -> To Workspace/1
  Demux/3 -> To Workspace2/1
  Demux/2 -> To Workspace1/1
  F/1 -> Demux/1

== system Parametrica/FIXED CHASSIS/BODY/FL HARDPOINTS/B forces sensing ==
  F : Inport
  Demux : Demux  Outputs=3
  To Workspace : ToWorkspace  VariableName=FL_B_Fx  SaveFormat=Timeseries  SampleTime=-1
  To Workspace1 : ToWorkspace  VariableName=FL_B_Fy  SaveFormat=Timeseries  SampleTime=-1
  To Workspace2 : ToWorkspace  VariableName=FL_B_Fz  SaveFormat=Timeseries  SampleTime=-1
  wires:
  Demux/1 -> To Workspace/1
  Demux/3 -> To Workspace2/1
  Demux/2 -> To Workspace1/1
  F/1 -> Demux/1

== system Parametrica/FIXED CHASSIS/BODY/FL HARDPOINTS/C forces sensing ==
  F : Inport
  Demux : Demux  Outputs=3
  To Workspace : ToWorkspace  VariableName=FL_C_Fx  SaveFormat=Timeseries  SampleTime=-1
  To Workspace1 : ToWorkspace  VariableName=FL_C_Fy  SaveFormat=Timeseries  SampleTime=-1
  To Workspace2 : ToWorkspace  VariableName=FL_C_Fz  SaveFormat=Timeseries  SampleTime=-1
  wires:
  Demux/1 -> To Workspace/1
  Demux/3 -> To Workspace2/1
  Demux/2 -> To Workspace1/1
  F/1 -> Demux/1

== system Parametrica/FIXED CHASSIS/BODY/FL HARDPOINTS/D forces sensing ==
  F : Inport
  Demux : Demux  Outputs=3
  To Workspace : ToWorkspace  VariableName=FL_D_Fx  SaveFormat=Timeseries  SampleTime=-1
  To Workspace1 : ToWorkspace  VariableName=FL_D_Fy  SaveFormat=Timeseries  SampleTime=-1
  To Workspace2 : ToWorkspace  VariableName=FL_D_Fz  SaveFormat=Timeseries  SampleTime=-1
  wires:
  Demux/1 -> To Workspace/1
  Demux/3 -> To Workspace2/1
  Demux/2 -> To Workspace1/1
  F/1 -> Demux/1

== system Parametrica/FIXED CHASSIS/BODY/FL HARDPOINTS/crank forces sensing ==
  F : Inport
  Demux : Demux  Outputs=3
  To Workspace : ToWorkspace  VariableName=FL_CRANK_Fx  SaveFormat=Timeseries  SampleTime=-1
  To Workspace1 : ToWorkspace  VariableName=FL_CRANK_Fy  SaveFormat=Timeseries  SampleTime=-1
  To Workspace2 : ToWorkspace  VariableName=FL_CRANK_Fz  SaveFormat=Timeseries  SampleTime=-1
  wires:
  Demux/1 -> To Workspace/1
  Demux/3 -> To Workspace2/1
  Demux/2 -> To Workspace1/1
  F/1 -> Demux/1

== system Parametrica/FIXED CHASSIS/BODY/FL HARDPOINTS/damper forces sensing ==
  F : Inport
  Demux : Demux  Outputs=3
  To Workspace : ToWorkspace  VariableName=FL_AMMO_Fx  SaveFormat=Timeseries  SampleTime=-1
  To Workspace1 : ToWorkspace  VariableName=FL_AMMO_Fy  SaveFormat=Timeseries  SampleTime=-1
  To Workspace2 : ToWorkspace  VariableName=FL_AMMO_Fz  SaveFormat=Timeseries  SampleTime=-1
  wires:
  Demux/1 -> To Workspace/1
  Demux/3 -> To Workspace2/1
  Demux/2 -> To Workspace1/1
  F/1 -> Demux/1

== system Parametrica/FIXED CHASSIS/BODY/FR HARDPOINTS/A forces sensing ==
  F : Inport
  Demux : Demux  Outputs=3
  To Workspace : ToWorkspace  VariableName=FR_A_Fx  SaveFormat=Timeseries  SampleTime=-1
  To Workspace1 : ToWorkspace  VariableName=FR_A_Fy  SaveFormat=Timeseries  SampleTime=-1
  To Workspace2 : ToWorkspace  VariableName=FR_A_Fz  SaveFormat=Timeseries  SampleTime=-1
  wires:
  Demux/1 -> To Workspace/1
  Demux/3 -> To Workspace2/1
  Demux/2 -> To Workspace1/1
  F/1 -> Demux/1

== system Parametrica/FIXED CHASSIS/BODY/FR HARDPOINTS/B forces sensing ==
  F : Inport
  Demux : Demux  Outputs=3
  To Workspace : ToWorkspace  VariableName=FR_B_Fx  SaveFormat=Timeseries  SampleTime=-1
  To Workspace1 : ToWorkspace  VariableName=FR_B_Fy  SaveFormat=Timeseries  SampleTime=-1
  To Workspace2 : ToWorkspace  VariableName=FR_B_Fz  SaveFormat=Timeseries  SampleTime=-1
  wires:
  Demux/1 -> To Workspace/1
  Demux/3 -> To Workspace2/1
  Demux/2 -> To Workspace1/1
  F/1 -> Demux/1

== system Parametrica/FIXED CHASSIS/BODY/FR HARDPOINTS/C forces sensing ==
  F : Inport
  Demux : Demux  Outputs=3
  To Workspace : ToWorkspace  VariableName=FR_C_Fx  SaveFormat=Timeseries  SampleTime=-1
  To Workspace1 : ToWorkspace  VariableName=FR_C_Fy  SaveFormat=Timeseries  SampleTime=-1
  To Workspace2 : ToWorkspace  VariableName=FR_C_Fz  SaveFormat=Timeseries  SampleTime=-1
  wires:
  Demux/1 -> To Workspace/1
  Demux/3 -> To Workspace2/1
  Demux/2 -> To Workspace1/1
  F/1 -> Demux/1

== system Parametrica/FIXED CHASSIS/BODY/FR HARDPOINTS/D forces sensing ==
  F : Inport
  Demux : Demux  Outputs=3
  To Workspace : ToWorkspace  VariableName=FR_D_Fx  SaveFormat=Timeseries  SampleTime=-1
  To Workspace1 : ToWorkspace  VariableName=FR_D_Fy  SaveFormat=Timeseries  SampleTime=-1
  To Workspace2 : ToWorkspace  VariableName=FR_D_Fz  SaveFormat=Timeseries  SampleTime=-1
  wires:
  Demux/1 -> To Workspace/1
  Demux/3 -> To Workspace2/1
  Demux/2 -> To Workspace1/1
  F/1 -> Demux/1

== system Parametrica/FIXED CHASSIS/BODY/FR HARDPOINTS/crank forces sensing ==
  F : Inport
  Demux : Demux  Outputs=3
  To Workspace : ToWorkspace  VariableName=FR_CRANK_Fx  SaveFormat=Timeseries  SampleTime=-1
  To Workspace1 : ToWorkspace  VariableName=FR_CRANK_Fy  SaveFormat=Timeseries  SampleTime=-1
  To Workspace2 : ToWorkspace  VariableName=FR_CRANK_Fz  SaveFormat=Timeseries  SampleTime=-1
  wires:
  Demux/1 -> To Workspace/1
  Demux/3 -> To Workspace2/1
  Demux/2 -> To Workspace1/1
  F/1 -> Demux/1

== system Parametrica/FIXED CHASSIS/BODY/FR HARDPOINTS/damper forces sensing ==
  F : Inport
  Demux : Demux  Outputs=3
  To Workspace : ToWorkspace  VariableName=FR_AMMO_Fx  SaveFormat=Timeseries  SampleTime=-1
  To Workspace1 : ToWorkspace  VariableName=FR_AMMO_Fy  SaveFormat=Timeseries  SampleTime=-1
  To Workspace2 : ToWorkspace  VariableName=FR_AMMO_Fz  SaveFormat=Timeseries  SampleTime=-1
  wires:
  Demux/1 -> To Workspace/1
  Demux/3 -> To Workspace2/1
  Demux/2 -> To Workspace1/1
  F/1 -> Demux/1

== system Parametrica/FIXED CHASSIS/BODY/RL HARDPOINTS/A forces sensing ==
  F : Inport
  Demux : Demux  Outputs=3
  To Workspace : ToWorkspace  VariableName=RL_A_Fx  SaveFormat=Timeseries  SampleTime=-1
  To Workspace1 : ToWorkspace  VariableName=RL_A_Fy  SaveFormat=Timeseries  SampleTime=-1
  To Workspace2 : ToWorkspace  VariableName=RL_A_Fz  SaveFormat=Timeseries  SampleTime=-1
  wires:
  Demux/1 -> To Workspace/1
  Demux/3 -> To Workspace2/1
  Demux/2 -> To Workspace1/1
  F/1 -> Demux/1

== system Parametrica/FIXED CHASSIS/BODY/RL HARDPOINTS/B forces sensing ==
  F : Inport
  Demux : Demux  Outputs=3
  To Workspace : ToWorkspace  VariableName=RL_B_Fx  SaveFormat=Timeseries  SampleTime=-1
  To Workspace1 : ToWorkspace  VariableName=RL_B_Fy  SaveFormat=Timeseries  SampleTime=-1
  To Workspace2 : ToWorkspace  VariableName=RL_B_Fz  SaveFormat=Timeseries  SampleTime=-1
  wires:
  Demux/1 -> To Workspace/1
  Demux/3 -> To Workspace2/1
  Demux/2 -> To Workspace1/1
  F/1 -> Demux/1

== system Parametrica/FIXED CHASSIS/BODY/RL HARDPOINTS/C forces sensing ==
  F : Inport
  Demux : Demux  Outputs=3
  To Workspace : ToWorkspace  VariableName=RL_C_Fx  SaveFormat=Timeseries  SampleTime=-1
  To Workspace1 : ToWorkspace  VariableName=RL_C_Fy  SaveFormat=Timeseries  SampleTime=-1
  To Workspace2 : ToWorkspace  VariableName=RL_C_Fz  SaveFormat=Timeseries  SampleTime=-1
  wires:
  Demux/1 -> To Workspace/1
  Demux/3 -> To Workspace2/1
  Demux/2 -> To Workspace1/1
  F/1 -> Demux/1

== system Parametrica/FIXED CHASSIS/BODY/RL HARDPOINTS/D forces sensing ==
  F : Inport
  Demux : Demux  Outputs=3
  To Workspace : ToWorkspace  VariableName=RL_D_Fx  SaveFormat=Timeseries  SampleTime=-1
  To Workspace1 : ToWorkspace  VariableName=RL_D_Fy  SaveFormat=Timeseries  SampleTime=-1
  To Workspace2 : ToWorkspace  VariableName=RL_D_Fz  SaveFormat=Timeseries  SampleTime=-1
  wires:
  Demux/1 -> To Workspace/1
  Demux/3 -> To Workspace2/1
  Demux/2 -> To Workspace1/1
  F/1 -> Demux/1

== system Parametrica/FIXED CHASSIS/BODY/RL HARDPOINTS/crank forces sensing ==
  F : Inport
  Demux : Demux  Outputs=3
  To Workspace : ToWorkspace  VariableName=RL_CRANK_Fx  SaveFormat=Timeseries  SampleTime=-1
  To Workspace1 : ToWorkspace  VariableName=RL_CRANK_Fy  SaveFormat=Timeseries  SampleTime=-1
  To Workspace2 : ToWorkspace  VariableName=RL_CRANK_Fz  SaveFormat=Timeseries  SampleTime=-1
  wires:
  Demux/1 -> To Workspace/1
  Demux/3 -> To Workspace2/1
  Demux/2 -> To Workspace1/1
  F/1 -> Demux/1

== system Parametrica/FIXED CHASSIS/BODY/RL HARDPOINTS/damper forces sensing ==
  F : Inport
  Demux : Demux  Outputs=3
  To Workspace : ToWorkspace  VariableName=RL_AMMO_Fx  SaveFormat=Timeseries  SampleTime=-1
  To Workspace1 : ToWorkspace  VariableName=RL_AMMO_Fy  SaveFormat=Timeseries  SampleTime=-1
  To Workspace2 : ToWorkspace  VariableName=RL_AMMO_Fz  SaveFormat=Timeseries  SampleTime=-1
  wires:
  Demux/1 -> To Workspace/1
  Demux/3 -> To Workspace2/1
  Demux/2 -> To Workspace1/1
  F/1 -> Demux/1

== system Parametrica/FIXED CHASSIS/BODY/RR HARDPOINTS/A forces sensing ==
  F : Inport
  Demux : Demux  Outputs=3
  To Workspace : ToWorkspace  VariableName=RR_A_Fx  SaveFormat=Timeseries  SampleTime=-1
  To Workspace1 : ToWorkspace  VariableName=RR_A_Fy  SaveFormat=Timeseries  SampleTime=-1
  To Workspace2 : ToWorkspace  VariableName=RR_A_Fz  SaveFormat=Timeseries  SampleTime=-1
  wires:
  Demux/1 -> To Workspace/1
  Demux/3 -> To Workspace2/1
  Demux/2 -> To Workspace1/1
  F/1 -> Demux/1

== system Parametrica/FIXED CHASSIS/BODY/RR HARDPOINTS/B forces sensing ==
  F : Inport
  Demux : Demux  Outputs=3
  To Workspace : ToWorkspace  VariableName=RR_B_Fx  SaveFormat=Timeseries  SampleTime=-1
  To Workspace1 : ToWorkspace  VariableName=RR_B_Fy  SaveFormat=Timeseries  SampleTime=-1
  To Workspace2 : ToWorkspace  VariableName=RR_B_Fz  SaveFormat=Timeseries  SampleTime=-1
  wires:
  Demux/1 -> To Workspace/1
  Demux/3 -> To Workspace2/1
  Demux/2 -> To Workspace1/1
  F/1 -> Demux/1

== system Parametrica/FIXED CHASSIS/BODY/RR HARDPOINTS/C forces sensing ==
  F : Inport
  Demux : Demux  Outputs=3
  To Workspace : ToWorkspace  VariableName=RR_C_Fx  SaveFormat=Timeseries  SampleTime=-1
  To Workspace1 : ToWorkspace  VariableName=RR_C_Fy  SaveFormat=Timeseries  SampleTime=-1
  To Workspace2 : ToWorkspace  VariableName=RR_C_Fz  SaveFormat=Timeseries  SampleTime=-1
  wires:
  Demux/1 -> To Workspace/1
  Demux/3 -> To Workspace2/1
  Demux/2 -> To Workspace1/1
  F/1 -> Demux/1

== system Parametrica/FIXED CHASSIS/BODY/RR HARDPOINTS/D forces sensing ==
  F : Inport
  Demux : Demux  Outputs=3
  To Workspace : ToWorkspace  VariableName=RR_D_Fx  SaveFormat=Timeseries  SampleTime=-1
  To Workspace1 : ToWorkspace  VariableName=RR_D_Fy  SaveFormat=Timeseries  SampleTime=-1
  To Workspace2 : ToWorkspace  VariableName=RR_D_Fz  SaveFormat=Timeseries  SampleTime=-1
  wires:
  Demux/1 -> To Workspace/1
  Demux/3 -> To Workspace2/1
  Demux/2 -> To Workspace1/1
  F/1 -> Demux/1

== system Parametrica/FIXED CHASSIS/BODY/RR HARDPOINTS/crank forces sensing ==
  F : Inport
  Demux : Demux  Outputs=3
  To Workspace : ToWorkspace  VariableName=RR_CRANK_Fx  SaveFormat=Timeseries  SampleTime=-1
  To Workspace1 : ToWorkspace  VariableName=RR_CRANK_Fy  SaveFormat=Timeseries  SampleTime=-1
  To Workspace2 : ToWorkspace  VariableName=RR_CRANK_Fz  SaveFormat=Timeseries  SampleTime=-1
  wires:
  Demux/1 -> To Workspace/1
  Demux/3 -> To Workspace2/1
  Demux/2 -> To Workspace1/1
  F/1 -> Demux/1

== system Parametrica/FIXED CHASSIS/BODY/RR HARDPOINTS/damper forces sensing ==
  F : Inport
  Demux : Demux  Outputs=3
  To Workspace : ToWorkspace  VariableName=RR_AMMO_Fx  SaveFormat=Timeseries  SampleTime=-1
  To Workspace1 : ToWorkspace  VariableName=RR_AMMO_Fy  SaveFormat=Timeseries  SampleTime=-1
  To Workspace2 : ToWorkspace  VariableName=RR_AMMO_Fz  SaveFormat=Timeseries  SampleTime=-1
  wires:
  Demux/1 -> To Workspace/1
  Demux/3 -> To Workspace2/1
  Demux/2 -> To Workspace1/1
  F/1 -> Demux/1

== system Parametrica/MOVING CHASSIS/ACTUATOR FL/ACTUATOR IN//OUT/Random sine waves ==
  Clock : Clock
  Constant : Constant  Value=Smi.general.random_harshness
  Constant1 : Constant  Value=-100
  Divide : Product  Inputs=*/
  First Order Hold : FirstOrderHold  InitialOutput=-100  ErrorTolerance=30  AllowContinuousInput=on
  Gain : Gain  Gain=100
  Random Source : dspsrcs4/Random Source  SrcType=Uniform  NormMethod=Ziggurat  CltLength=12  MinVal=-Smi.general.random_amplitude*0.5  MaxVal=Smi.general.random_amplitude*0.5  MeanVal=0  VarVal=1  RepMode=Not repeatable  rawSeed=1  IsInherit=off  SampMode=Discrete  SampTime=0.05  SampFrame=1  DataType=Double  OutComplex=Real  OutputFrames=off
  Rate Transition : RateTransition  OutPortSampleTime=0
  Sum : Sum  Inputs=|+-
  Switch : Switch  Criteria=u2 ~= 0
  Varying Lowpass Filter : cstblocks/Linear Parameter Varying/Varying Lowpass Filter  N=5
  f : Outport
  wires:
  Constant/1 -> Varying Lowpass Filter/2
  Random Source/1 -> Rate Transition/1
  Divide/1 -> Gain/1
  Gain/1 -> Sum/2
  Varying Lowpass Filter/1 -> First Order Hold/1
  First Order Hold/1 -> Sum/1
  Clock/1 -> Divide/2, Switch/2, Divide/1
  Sum/1 -> Switch/1
  Constant1/1 -> Switch/3
  Switch/1 -> f/1
  Rate Transition/1 -> Varying Lowpass Filter/1

== system Parametrica/MOVING CHASSIS/ACTUATOR FR/ACTUATOR IN//OUT/Random sine waves ==
  Clock : Clock
  Constant : Constant  Value=Smi.general.random_harshness
  Constant1 : Constant  Value=-100
  Divide : Product  Inputs=*/
  First Order Hold : FirstOrderHold  InitialOutput=-100  ErrorTolerance=30  AllowContinuousInput=on
  Gain : Gain  Gain=100
  Random Source : dspsrcs4/Random Source  SrcType=Uniform  NormMethod=Ziggurat  CltLength=12  MinVal=-Smi.general.random_amplitude*0.5  MaxVal=Smi.general.random_amplitude*0.5  MeanVal=0  VarVal=1  RepMode=Not repeatable  rawSeed=1  IsInherit=off  SampMode=Discrete  SampTime=0.05  SampFrame=1  DataType=Double  OutComplex=Real  OutputFrames=off
  Rate Transition : RateTransition  OutPortSampleTime=0
  Sum : Sum  Inputs=|+-
  Switch : Switch  Criteria=u2 ~= 0
  Varying Lowpass Filter : cstblocks/Linear Parameter Varying/Varying Lowpass Filter  N=5
  f : Outport
  wires:
  Constant/1 -> Varying Lowpass Filter/2
  Random Source/1 -> Rate Transition/1
  Divide/1 -> Gain/1
  Gain/1 -> Sum/2
  Varying Lowpass Filter/1 -> First Order Hold/1
  First Order Hold/1 -> Sum/1
  Clock/1 -> Divide/2, Switch/2, Divide/1
  Sum/1 -> Switch/1
  Constant1/1 -> Switch/3
  Switch/1 -> f/1
  Rate Transition/1 -> Varying Lowpass Filter/1

== system Parametrica/MOVING CHASSIS/ACTUATOR RL/ACTUATOR IN//OUT/Random sine waves ==
  Clock : Clock
  Constant : Constant  Value=Smi.general.random_harshness
  Constant1 : Constant  Value=-100
  Divide : Product  Inputs=*/
  First Order Hold : FirstOrderHold  InitialOutput=-100  ErrorTolerance=30  AllowContinuousInput=on
  Gain : Gain  Gain=100
  Random Source : dspsrcs4/Random Source  SrcType=Uniform  NormMethod=Ziggurat  CltLength=12  MinVal=-Smi.general.random_amplitude*0.5  MaxVal=Smi.general.random_amplitude*0.5  MeanVal=0  VarVal=1  RepMode=Not repeatable  rawSeed=1  IsInherit=off  SampMode=Discrete  SampTime=0.05  SampFrame=1  DataType=Double  OutComplex=Real  OutputFrames=off
  Rate Transition : RateTransition  OutPortSampleTime=0
  Sum : Sum  Inputs=|+-
  Switch : Switch  Criteria=u2 ~= 0
  Varying Lowpass Filter : cstblocks/Linear Parameter Varying/Varying Lowpass Filter  N=5
  f : Outport
  wires:
  Constant/1 -> Varying Lowpass Filter/2
  Random Source/1 -> Rate Transition/1
  Divide/1 -> Gain/1
  Gain/1 -> Sum/2
  Varying Lowpass Filter/1 -> First Order Hold/1
  First Order Hold/1 -> Sum/1
  Clock/1 -> Divide/2, Switch/2, Divide/1
  Sum/1 -> Switch/1
  Constant1/1 -> Switch/3
  Switch/1 -> f/1
  Rate Transition/1 -> Varying Lowpass Filter/1
